simulink model "Observateur_step1"  (R2017a)
settings: Solver=VariableStepAuto  StartTime=0.0  StopTime=2  RelTol=1e-3
undefined symbols (not defined in the file): A, Ao, B, Bo, C, Co, u0, uf, x0, xo0
settings Model: Creator=Alex  LastModifiedBy=Alex
settings DataIOCC: ReturnWorkspaceOutputs=on
settings SFSimCC: SimUseLocalCustomCode=on
settings RTWCC: RTWUseLocalCustomCode=on

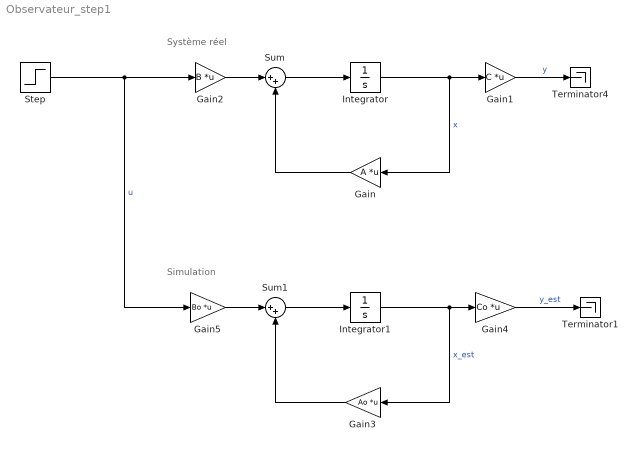
== system Observateur_step1 ==
  note: Système réel
  note: Simulation
  Gain : Gain  Gain=A  Multiplication=Matrix(K*u)
  Gain1 : Gain  Gain=C  Multiplication=Matrix(K*u)
  Gain2 : Gain  Gain=B  Multiplication=Matrix(K*u)
  Gain3 : Gain  Gain=Ao  Multiplication=Matrix(K*u)
  Gain4 : Gain  Gain=Co  Multiplication=Matrix(K*u)
  Gain5 : Gain  Gain=Bo  Multiplication=Matrix(K*u)
  Integrator : Integrator  InitialCondition=x0
      settings: AttributesFormatString=Conditions intiales %<InitialCondition>
  Integrator1 : Integrator  InitialCondition=xo0
      settings: AttributesFormatString=Conditions intiales %<InitialCondition>
  Step : Step  Before=u0  After=uf  SampleTime=0
  Sum : Sum  Inputs=|++
  Sum1 : Sum  Inputs=|++
  Terminator1 : Terminator
  Terminator4 : Terminator
  wires:
  Sum/1 -> Integrator/1
  Gain/1 -> Sum/2
  Integrator/1 -> Gain1/1, Gain/1  "x"
  Gain1/1 -> Terminator4/1  "y"
  Gain2/1 -> Sum/1
  Step/1 -> Gain5/1, Gain2/1  "u"
  Gain5/1 -> Sum1/1
  Integrator1/1 -> Gain3/1, Gain4/1  "x_est"
  Gain3/1 -> Sum1/2
  Sum1/1 -> Integrator1/1
  Gain4/1 -> Terminator1/1  "y_est"
